simulink model "RLUb"  (R2018b)
settings: Solver=VariableStepAuto  StartTime=0.0  StopTime=15e-3  RelTol=1e-6  EnableMultiTasking=on
InitFcn:
  | RLUb_init
values from neighbouring files (symbols this model uses):
  D0 = Uout0 / Udc    [pmsm_control_init.m]
  Deadtime = 0e-6    (= 0)    [pmsm_control_init.m]
  dt = 50e-9    (= 5e-08)    [pmsm_init.m]
  fsw = 10e3    (= 10000)    [pmsm_control_init.m]
  I_FS = IabcFS / 0.8    [pmsm_control_init.m]
  L = Ld    [pmsm_control_init.m]    (also in pmsm_init.m = [Ld Lq])
  R = 18e-3    (= 0.018)    [pmsm_init.m]
  SampleMode = 1    [pmsm_control_init.m]
  U_FS = Udc / 0.8    [pmsm_control_init.m]
  Ub = Udc / 2    [pmsm_control_init.m]
  Udc = 300    [pmsm_init.m]
undefined symbols (not defined in the file or in its folder): A_I, A_P
libraries: powerlib x9, simulink x7
settings Model: ModifiedByFormat=The MathWorks Inc.  Creator=The MathWorks, Inc.  LastModifiedBy=The MathWorks Inc.
settings DataIOCC: LimitDataPoints=on  SaveFormat=Array  SaveOutput=off  SaveTime=off
settings OptimizationCC: ExpressionDepthLimit=2147483647  LifeSpan=1
settings DebuggingCC: MergeDetectMultiDrivingBlocksExec=none  SolverPrmCheckMsg=warning  FcnCallInpInsideContextMsg=warning  StateNameClashWarn=warning  SFUnexpectedBacktrackingDiag=warning  SFNoUnconditionalDefaultTransitionDiag=warning  SFExecutionAtInitializationDiag=none
settings HardwareCC: ProdBitPerPointer=32  ProdBitPerSizeT=32  ProdBitPerPtrDiffT=32  ProdLargestAtomicFloat=None  ProdIntDivRoundTo=Undefined  ProdEndianess=Unspecified  ProdWordSize=32  ProdHWDeviceType=32-bit Generic
settings ModelReferenceCC: PropagateSignalLabelsOutOfModel=off
settings SFSimCC: SimUseLocalCustomCode=off
settings RTWCC: RTWUseLocalCustomCode=off
settings CodeAppCC: StateflowObjectComments=on
settings GRTTargetCC: TargetLangStandard=C89/C90 (ANSI)  GeneratePreprocessorConditionals=Disable all  CombineOutputUpdateFcns=off  GRTInterface=on
settings ConfigComp: CovMetricSettings=dw  CovHtmlReporting=on  CovSaveCumulativeToWorkspaceVar=on  CovSaveSingleToWorkspaceVar=on  CovExternalEMLEnable=off  CovSFcnEnable=off

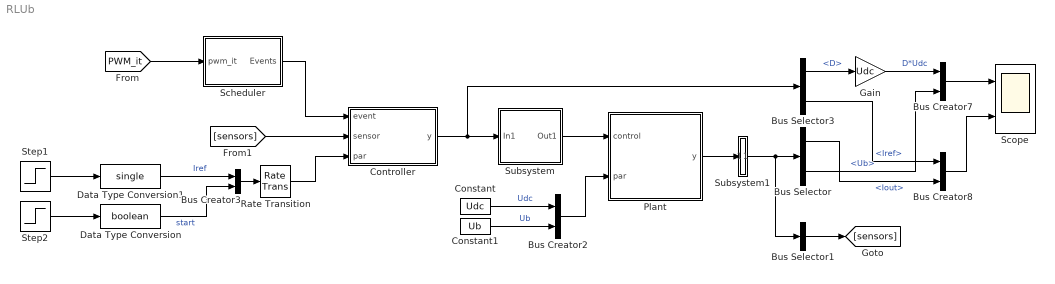
== system RLUb ==
  Bus Creator{2..3,7..8} (4 alike) : BusCreator  Inputs=2
  Bus Selector : BusSelector  OutputSignals=Iout,Ub
  Bus Selector1 : BusSelector  OutputSignals=Iout,Udc,Ub  OutputAsBus=on
  Bus Selector3 : BusSelector  OutputSignals=D,Iref
  Constant : Constant  Value=Udc  SampleTime=-1
  Constant1 : Constant  Value=Ub  SampleTime=-1
  Controller : Subsystem
  Data Type Conversion : DataTypeConversion  OutDataTypeStr=boolean
  Data Type Conversion1 : DataTypeConversion  OutDataTypeStr=single
  Gain : Gain  Gain=Udc
  Plant : Subsystem  Variant=on
  Rate Transition : RateTransition  Integrity=off  Deterministic=off
  Scheduler : Subsystem
  Scope : Scope  NumInputPorts=2
  Step1 : Step  Time=[7e-3]  After=10  SampleTime=0
  Step2 : Step  Time=[2e-3]  After=1e-3  SampleTime=0
  Subsystem : Subsystem
  Subsystem1 : Subsystem
  wires:
  Constant/1 -> Bus Creator2/1  "Udc"
  Constant1/1 -> Bus Creator2/2  "Ub"
  Bus Selector1/1 -> [sensors]
  Controller/1(y) -> Bus Selector3/1, Subsystem/1(In1)
  Bus Selector3/1 -> Gain/1  "<D>"
  Gain/1 -> Bus Creator7/1  "D*Udc"
  Bus Selector3/2 -> Bus Creator8/1  "<Iref>"
  Bus Selector/1 -> Bus Creator8/2  "<Iout>"
  Bus Creator7/1 -> Scope/1
  Bus Creator8/1 -> Scope/2
  Step1/1 -> Data Type Conversion1/1
  Scheduler/1(Events) -> Controller/1(event)
  Step2/1 -> Data Type Conversion/1
  Data Type Conversion/1 -> Bus Creator3/2  "start"
  Data Type Conversion1/1 -> Bus Creator3/1  "Iref"
  Bus Creator3/1 -> Rate Transition/1
  Plant/1(y) -> Subsystem1/1(In1)
  Bus Creator2/1 -> Plant/2(par)
  [sensors] -> Controller/2(sensor)
  Bus Selector/2 -> Bus Creator7/2  "<Ub>"
  Subsystem1/1(Out1) -> Bus Selector1/1, Bus Selector/1
  Rate Transition/1 -> Controller/3(par)
  [PWM_it] -> Scheduler/1(pwm_it)
  Subsystem/1(Out1) -> Plant/1(control)

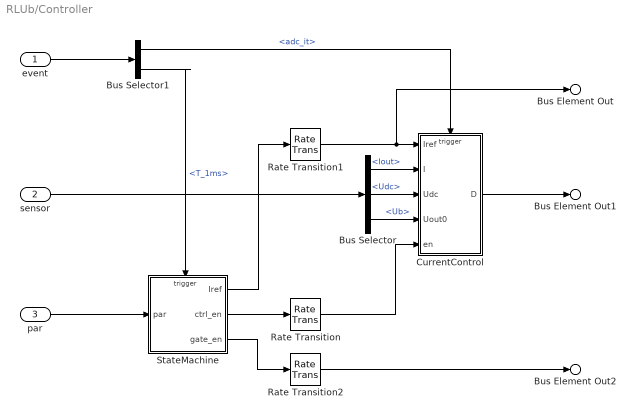
== system RLUb/Controller ==
  event : Inport
  sensor : Inport  Port=2
  par : Inport  Port=3
  Bus Selector : BusSelector  OutputSignals=Iout,Udc,Ub
  Bus Selector1 : BusSelector  OutputSignals=interrupts.adc_it,timers.T_1ms
  CurrentControl : Subsystem
  Rate Transition : RateTransition  Integrity=off  Deterministic=off
  Rate Transition1 : RateTransition  Integrity=off  Deterministic=off
  Rate Transition2 : RateTransition  Integrity=off  Deterministic=off
  StateMachine : Subsystem  TreatAsAtomicUnit=on
  Bus Element Out : Outport  PortName=y  Element=Iref
  Bus Element Out1 : Outport  PortName=y  Element=D
  Bus Element Out2 : Outport  PortName=y  Element=gate_en
  wires:
  StateMachine/1(Iref) -> Rate Transition1/1
  Rate Transition/1 -> CurrentControl/5(en)
  sensor/1 -> Bus Selector/1
  Bus Selector/1 -> CurrentControl/2(I)  "<Iout>"
  Bus Selector/2 -> CurrentControl/3(Udc)  "<Udc>"
  event/1 -> Bus Selector1/1
  Bus Selector1/1 -> CurrentControl/Trigger  "<adc_it>"
  CurrentControl/1(D) -> Bus Element Out1/1
  Bus Selector/3 -> CurrentControl/4(Uout0)  "<Ub>"
  Bus Selector1/2 -> StateMachine/Trigger  "<T_1ms>"
  StateMachine/2(ctrl_en) -> Rate Transition/1
  par/1 -> StateMachine/1(par)
  Rate Transition1/1 -> Bus Element Out/1, CurrentControl/1(Iref)
  StateMachine/3(gate_en) -> Rate Transition2/1
  Rate Transition2/1 -> Bus Element Out2/1

== system RLUb/Plant ==
  note: 1) Add Subsystem or Model blocks as valid variant choices.
      | 2) You cannot connect blocks at this level. At simulation, connectivity is automatically
      | determined, based on the active variant and port name matching.
  control : Inport
  par : Inport  Port=2
  RLUb_CT : Subsystem  VariantControl=PlantVariant == 11
  RLUb_DT : Subsystem  VariantControl=PlantVariant == 12
  RLUb_DTFX : Subsystem  VariantControl=PlantVariant == 13
  RLUb_SimPower : Subsystem  VariantControl=PlantVariant == 10
  y : Outport

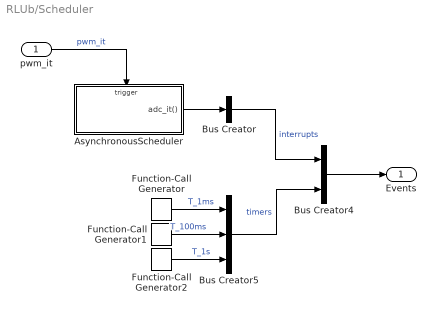
== system RLUb/Scheduler ==
  pwm_it : Inport
  AsynchronousScheduler : Stateflow chart  TreatAsAtomicUnit=on
      settings: RTWMemSecFuncInitTerm=Default  RTWMemSecFuncExecute=Default
  Bus Creator : BusCreator  Inputs=1
  Bus Creator4 : BusCreator  Inputs=2
  Bus Creator5 : BusCreator  Inputs=3
  Function-Call Generator : simulink/Ports & Subsystems/Function-Call Generator  sample_time=1e-3  numberOfIterations=1
  Function-Call Generator1 : simulink/Ports & Subsystems/Function-Call Generator  sample_time=100e-3  numberOfIterations=1
  Function-Call Generator2 : simulink/Ports & Subsystems/Function-Call Generator  sample_time=1  numberOfIterations=1
  Events : Outport
  wires:
  Bus Creator5/1 -> Bus Creator4/2  "timers"
  Function-Call Generator2/1 -> Bus Creator5/3  "T_1s"
  Bus Creator/1 -> Bus Creator4/1  "interrupts"
  pwm_it/1 -> AsynchronousScheduler/Trigger  "pwm_it"
  AsynchronousScheduler/1(adc_it()) -> Bus Creator/1
  Bus Creator4/1 -> Events/1
  Function-Call Generator1/1 -> Bus Creator5/2  "T_100ms"
  Function-Call Generator/1 -> Bus Creator5/1  "T_1ms"

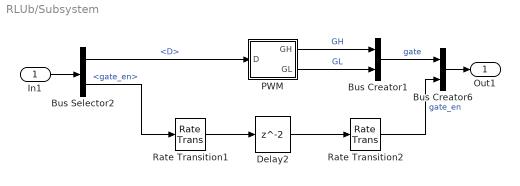
== system RLUb/Subsystem ==
  In1 : Inport
  Bus Creator1 : BusCreator  Inputs=2
  Bus Creator6 : BusCreator  Inputs=2
  Bus Selector2 : BusSelector  OutputSignals=D,gate_en
  Delay2 : Delay  InitialCondition=0
  PWM : Subsystem
  Rate Transition1 : RateTransition  Integrity=off  Deterministic=off  OutPortSampleTime=1e-3
  Rate Transition2 : RateTransition  Integrity=off  Deterministic=off
  Out1 : Outport
  wires:
  Rate Transition2/1 -> Bus Creator6/2  "gate_en"
  PWM/1(GH) -> Bus Creator1/1  "GH"
  Rate Transition1/1 -> Delay2/1
  Bus Selector2/1 -> PWM/1(D)  "<D>"
  Bus Selector2/2 -> Rate Transition1/1  "<gate_en>"
  Delay2/1 -> Rate Transition2/1
  In1/1 -> Bus Selector2/1
  PWM/2(GL) -> Bus Creator1/2  "GL"
  Bus Creator6/1 -> Out1/1
  Bus Creator1/1 -> Bus Creator6/1  "gate"

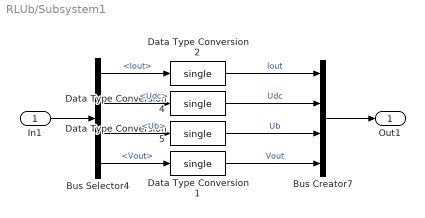
== system RLUb/Subsystem1 ==
  In1 : Inport
  Bus Creator7 : BusCreator  Inputs=4
  Bus Selector4 : BusSelector  OutputSignals=Iout,Udc,Ub,Vout
  Data Type Conversion{1..2,4..5} (4 alike) : DataTypeConversion  OutDataTypeStr=single
  Out1 : Outport
  wires:
  Data Type Conversion4/1 -> Bus Creator7/2  "Udc"
  Data Type Conversion2/1 -> Bus Creator7/1  "Iout"
  Bus Selector4/3 -> Data Type Conversion5/1  "<Ub>"
  Data Type Conversion5/1 -> Bus Creator7/3  "Ub"
  Bus Selector4/2 -> Data Type Conversion4/1  "<Udc>"
  Bus Selector4/1 -> Data Type Conversion2/1  "<Iout>"
  In1/1 -> Bus Selector4/1
  Bus Creator7/1 -> Out1/1
  Bus Selector4/4 -> Data Type Conversion1/1  "<Vout>"
  Data Type Conversion1/1 -> Bus Creator7/4  "Vout"

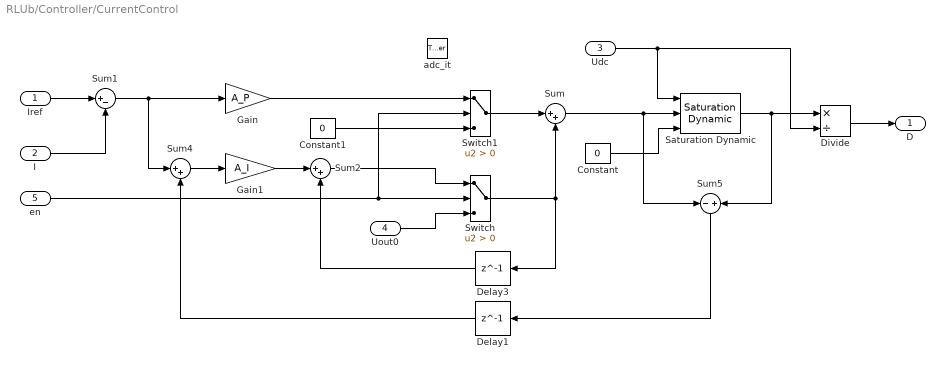
== system RLUb/Controller/CurrentControl ==
  Iref : Inport
  I : Inport  Port=2
  Udc : Inport  Port=3
  Uout0 : Inport  Port=4
  en : Inport  Port=5
  adc_it : TriggerPort  TriggerType=function-call  VariantControl=Variant  PortDimensions=1
  Constant : Constant  Value=0  OutDataTypeStr=Inherit: Inherit via back propagation  SampleTime=-1
  Constant1 : Constant  Value=0  OutDataTypeStr=Inherit: Inherit via back propagation  SampleTime=-1
  Delay1 : Delay  DelayLength=1  InitialCondition=0
  Delay3 : Delay  DelayLength=1  InitialCondition=0
  Divide : Product  Inputs=*/
  Gain : Gain  Gain=A_P
  Gain1 : Gain  Gain=A_I
  Saturation Dynamic : simulink/Discontinuities/Saturation Dynamic  OutMin=[]  OutMax=[]  OutDataTypeStr=Inherit: Same as second input  OutDataType=fixdt(1, 16)  OutScaling=2^-10  DoSatur=off
  Sum : Sum  Inputs=|++
  Sum1 : Sum  Inputs=|+-
  Sum2 : Sum  Inputs=|++
  Sum4 : Sum  Inputs=|++
  Sum5 : Sum  Inputs=-|+
  Switch : Switch  Criteria=u2 > Threshold
  Switch1 : Switch  Criteria=u2 > Threshold
  D : Outport
  wires:
  Divide/1 -> D/1
  Saturation Dynamic/1 -> Sum5/2, Divide/1
  Constant/1 -> Saturation Dynamic/3
  I/1 -> Sum1/2
  Udc/1 -> Divide/2, Saturation Dynamic/1
  Gain1/1 -> Sum2/1
  Iref/1 -> Sum1/1
  Uout0/1 -> Switch/3
  Sum4/1 -> Gain1/1
  Switch/1 -> Sum/2, Delay3/1
  Sum/1 -> Sum5/1, Saturation Dynamic/2
  Sum2/1 -> Switch/1
  Sum5/1 -> Delay1/1
  Sum1/1 -> Gain/1, Sum4/1
  Delay3/1 -> Sum2/2
  Delay1/1 -> Sum4/2
  Gain/1 -> Switch1/1
  Constant1/1 -> Switch1/3
  Switch1/1 -> Sum/1
  en/1 -> Switch1/2, Switch/2

== system RLUb/Controller/StateMachine ==
  par : Inport
  timer_1ms : TriggerPort  TriggerType=function-call  VariantControl=Variant
  Bus Selector2 : BusSelector  OutputSignals=Iref,start
  Delay1 : Delay  DelayLength=1  InitialCondition=0
  Delay2 : Delay  InitialCondition=0
  Iref : Outport
  ctrl_en : Outport  Port=2
  gate_en : Outport  Port=3
  wires:
  par/1 -> Delay1/1
  Bus Selector2/2 -> Delay2/1, gate_en/1  "<start>"
  Bus Selector2/1 -> Iref/1  "<Iref>"
  Delay1/1 -> Bus Selector2/1
  Delay2/1 -> ctrl_en/1

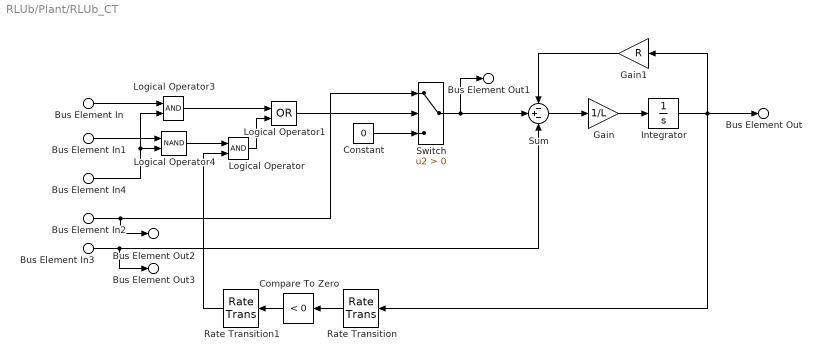
== system RLUb/Plant/RLUb_CT ==
  Bus Element In : Inport  PortName=control  Element=gate.GH
  Bus Element In1 : Inport  PortName=control  Element=gate.GL
  Bus Element In4 : Inport  PortName=control  Element=gate_en
  Bus Element In2 : Inport  Port=2  PortName=par  Element=Udc
  Bus Element In3 : Inport  Port=2  PortName=par  Element=Ub
  Compare To Zero : simulink/Logic and Bit Operations/Compare To Zero  relop=<  OutDataTypeStr=boolean
  Constant : Constant  Value=0  SampleTime=-1
  Gain : Gain  Gain=1/L
  Gain1 : Gain  Gain=R
  Integrator : Integrator
  Logical Operator : Logic  IconShape=distinctive  AllPortsSameDT=off  OutDataTypeStr=boolean
  Logical Operator1 : Logic  Operator=OR  IconShape=distinctive  AllPortsSameDT=off  OutDataTypeStr=boolean
  Logical Operator3 : Logic  IconShape=distinctive  AllPortsSameDT=off  OutDataTypeStr=boolean
  Logical Operator4 : Logic  Operator=NAND  IconShape=distinctive  AllPortsSameDT=off  OutDataTypeStr=boolean
  Rate Transition : RateTransition  OutPortSampleTime=1e-7
  Rate Transition1 : RateTransition
  Sum : Sum  Inputs=-+-
  Switch : Switch  Criteria=u2 > Threshold
  Bus Element Out : Outport  PortName=y  Element=Iout
  Bus Element Out1 : Outport  PortName=y  Element=Vout
  Bus Element Out2 : Outport  PortName=y  Element=Udc
  Bus Element Out3 : Outport  PortName=y  Element=Ub
  wires:
  Rate Transition/1 -> Compare To Zero/1
  Integrator/1 -> Rate Transition/1, Bus Element Out/1, Gain1/1
  Switch/1 -> Bus Element Out1/1, Sum/2
  Sum/1 -> Gain/1
  Gain/1 -> Integrator/1
  Gain1/1 -> Sum/1
  Bus Element In3/1 -> Bus Element Out3/1, Sum/3
  Bus Element In2/1 -> Bus Element Out2/1, Switch/1
  Constant/1 -> Switch/3
  Logical Operator3/1 -> Logical Operator1/1
  Logical Operator/1 -> Logical Operator1/2
  Logical Operator1/1 -> Switch/2
  Logical Operator4/1 -> Logical Operator/1
  Compare To Zero/1 -> Rate Transition1/1
  Rate Transition1/1 -> Logical Operator/2
  Bus Element In/1 -> Logical Operator3/1
  Bus Element In1/1 -> Logical Operator4/1
  Bus Element In4/1 -> Logical Operator3/2, Logical Operator4/2

== system RLUb/Plant/RLUb_DT ==
  control : Inport
  par : Inport  Port=2
  RLUb_DT : Subsystem  VariantControl=PlantVariant == 12
  Rate Transition : RateTransition  OutPortSampleTime=dt
  Rate Transition1 : RateTransition  OutPortSampleTime=dt
  Rate Transition2 : RateTransition
  y : Outport
  wires:
  control/1 -> Rate Transition/1
  RLUb_DT/1(y) -> Rate Transition2/1
  par/1 -> Rate Transition1/1
  Rate Transition/1 -> RLUb_DT/1(control)
  Rate Transition1/1 -> RLUb_DT/2(par)
  Rate Transition2/1 -> y/1

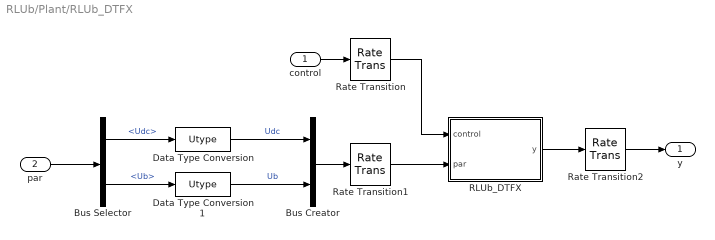
== system RLUb/Plant/RLUb_DTFX ==
  control : Inport
  par : Inport  Port=2
  Bus Creator : BusCreator  Inputs=2
  Bus Selector : BusSelector  OutputSignals=Udc,Ub
  Data Type Conversion : DataTypeConversion  OutDataTypeStr=Utype
  Data Type Conversion1 : DataTypeConversion  OutDataTypeStr=Utype
  RLUb_DTFX : Subsystem  VariantControl=PlantVariant == 12
  Rate Transition : RateTransition  OutPortSampleTime=dt
  Rate Transition1 : RateTransition  OutPortSampleTime=dt
  Rate Transition2 : RateTransition
  y : Outport
  wires:
  Rate Transition1/1 -> RLUb_DTFX/2(par)
  Rate Transition/1 -> RLUb_DTFX/1(control)
  RLUb_DTFX/1(y) -> Rate Transition2/1
  control/1 -> Rate Transition/1
  Rate Transition2/1 -> y/1
  Bus Creator/1 -> Rate Transition1/1
  Bus Selector/2 -> Data Type Conversion1/1  "<Ub>"
  par/1 -> Bus Selector/1
  Data Type Conversion/1 -> Bus Creator/1  "Udc"
  Bus Selector/1 -> Data Type Conversion/1  "<Udc>"
  Data Type Conversion1/1 -> Bus Creator/2  "Ub"

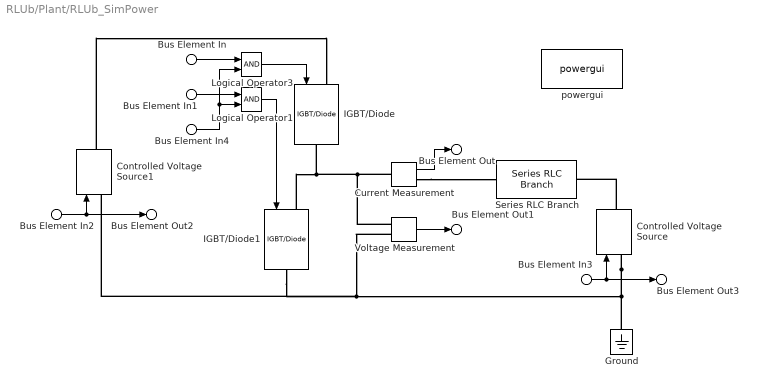
== system RLUb/Plant/RLUb_SimPower ==
  Bus Element In : Inport  PortName=control  Element=gate.GH
  Bus Element In1 : Inport  PortName=control  Element=gate.GL
  Bus Element In4 : Inport  PortName=control  Element=gate_en
  Bus Element In2 : Inport  Port=2  PortName=par  Element=Udc
  Bus Element In3 : Inport  Port=2  PortName=par  Element=Ub
  Controlled Voltage Source : powerlib/Electrical Sources/Controlled Voltage Source  Initialize=off  Source_Type=DC  Amplitude=0  Phase=0  Frequency=0  Measurements=None
  Controlled Voltage Source1 : powerlib/Electrical Sources/Controlled Voltage Source  Initialize=off  Source_Type=DC  Amplitude=0  Phase=0  Frequency=0  Measurements=None
  Current Measurement : powerlib/Measurements/Current Measurement  PhasorSimulation=off  OutputType=Complex  PSBequivalent=0
  Ground : powerlib/Elements/Ground  LConnTagsString=a
  IGBT/Diode : powerlib/Power Electronics/IGBT//Diode  Ron=1e-3  Rs=1e5  Cs=inf  Measurements=off
  IGBT/Diode1 : powerlib/Power Electronics/IGBT//Diode  Ron=1e-3  Rs=1e5  Cs=inf  Measurements=off
  Logical Operator1 : Logic  IconShape=distinctive  AllPortsSameDT=off  OutDataTypeStr=boolean
  Logical Operator3 : Logic  IconShape=distinctive  AllPortsSameDT=off  OutDataTypeStr=boolean
  Series RLC Branch : powerlib/Elements/Series RLC Branch  LConnTagsString=__new0  RConnTagsString=__new0  BranchType=RL  Resistance=R  Inductance=L  SetiL0=off  InitialCurrent=0  Capacitance=1e-6  Setx0=off  InitialVoltage=0  Measurements=None
  Voltage Measurement : powerlib/Measurements/Voltage Measurement  PhasorSimulation=off  OutputType=Complex  PSBequivalent=0
  powergui : powerlib/powergui  Priority=1  SimulationMode=Continuous  SampleTime=50e-6  frequency=60  Iterations=50  frequencyindice=0  Pbase=100e6  ErrMax=1e-4  UnitsV=kV  UnitsW=MW  buscounter=0  FunctionMessages=off  echomessages=off  EnableUseOfTLC=off  CurrentSourceSwitches=off  DisableSnubberDevices=off  DisableRonSwitches=off  DisableVfSwitches=off  DisplayEquations=off  SolverType=Tustin/Backward Euler (TBE)  Interpol=off  ExternalGateDelay=off  methode=off  Ts=100  x0status=blocks  SPID=on  SwTol=0  HookPort=off  RestoreLinks=warning  ResistiveCurrentMeasurement=off  Frange=[0:2:500]  Ylog=off  Xlog=on  ShowGrid=off  save=off  variable=ZData  structure=0  ZoomFFT=off  StartTime=0.0  cycles=1  DisplayStyle=1  fundamental=60  FreqAxis=off  MaxFrequency=1000  frequencyindicesteady=1  RmsSteady=1  display=off
  Bus Element Out : Outport  PortName=y  Element=Iout
  Bus Element Out1 : Outport  PortName=y  Element=Vout
  Bus Element Out2 : Outport  PortName=y  Element=Udc
  Bus Element Out3 : Outport  PortName=y  Element=Ub
  wires:
  Bus Element In2/1 -> Bus Element Out2/1, Controlled Voltage Source1/1
  Voltage Measurement/1 -> Bus Element Out1/1
  Current Measurement/1 -> Bus Element Out/1
  Bus Element In3/1 -> Controlled Voltage Source/1, Bus Element Out3/1
  Logical Operator1/1 -> IGBT/Diode1/1
  Logical Operator3/1 -> IGBT/Diode/1
  Bus Element In/1 -> Logical Operator3/1
  Bus Element In1/1 -> Logical Operator1/1
  Bus Element In4/1 -> Logical Operator1/2, Logical Operator3/2
  connections:
  Voltage Measurement/LConn1 -- Current Measurement/LConn1 -- IGBT/Diode1/LConn1 -- IGBT/Diode/RConn1
  Controlled Voltage Source/RConn1 -- Series RLC Branch/RConn1
  Controlled Voltage Source/LConn1 -- Ground/LConn1 -- Controlled Voltage Source1/LConn1 -- IGBT/Diode1/RConn1 -- Voltage Measurement/LConn2
  Controlled Voltage Source1/RConn1 -- IGBT/Diode/LConn1
  Current Measurement/RConn1 -- Series RLC Branch/LConn1

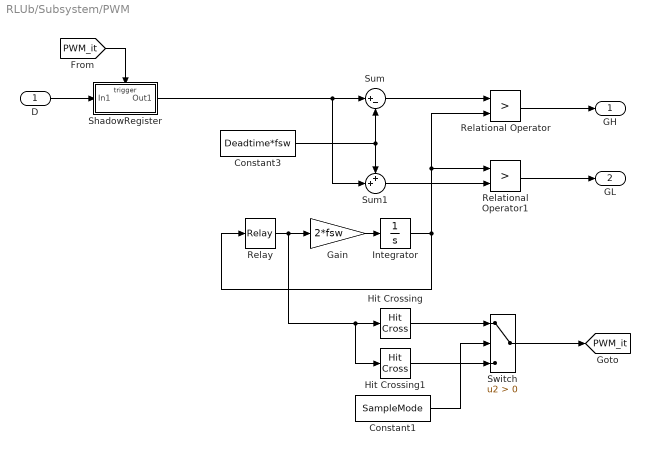
== system RLUb/Subsystem/PWM ==
  D : Inport
  Constant1 : Constant  Value=SampleMode  SampleTime=-1
  Constant3 : Constant  Value=Deadtime*fsw  SampleTime=-1
  Gain : Gain  Gain=2*fsw
  Hit Crossing : HitCross
  Hit Crossing1 : HitCross  HitCrossingDirection=rising
  Integrator : Integrator
  Relational Operator : RelationalOperator  Operator=>  OutDataTypeStr=boolean  RndMeth=Simplest
  Relational Operator1 : RelationalOperator  Operator=>  OutDataTypeStr=boolean  RndMeth=Simplest
  Relay : Relay  OnSwitchValue=1  OffSwitchValue=0  OnOutputValue=-1  OffOutputValue=1
  ShadowRegister : Subsystem
  Sum : Sum  Inputs=|+-
  Sum1 : Sum  Inputs=++|
  Switch : Switch  Criteria=u2 > Threshold
  GH : Outport
  GL : Outport  Port=2
  tag scope: PWM_it=global
  wires:
  Integrator/1 -> Relational Operator/2, Relational Operator1/1, Relay/1
  Gain/1 -> Integrator/1
  Relational Operator1/1 -> GL/1
  Relay/1 -> Hit Crossing1/1, Hit Crossing/1, Gain/1
  Constant3/1 -> Sum1/1, Sum/2
  Relational Operator/1 -> GH/1
  Sum1/1 -> Relational Operator1/2
  Sum/1 -> Relational Operator/1
  ShadowRegister/1(Out1) -> Sum1/2, Sum/1
  Hit Crossing/1 -> Switch/1
  Switch/1 -> [PWM_it]
  Hit Crossing1/1 -> Switch/3
  Constant1/1 -> Switch/2
  D/1 -> ShadowRegister/1(In1)
  [PWM_it] -> ShadowRegister/Trigger

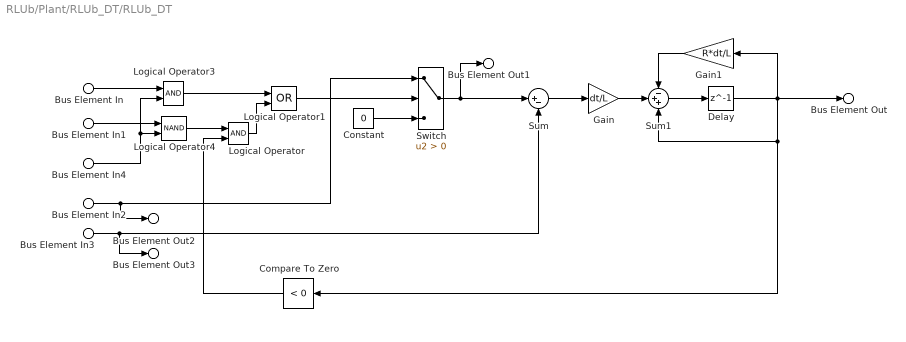
== system RLUb/Plant/RLUb_DT/RLUb_DT ==
  Bus Element In : Inport  PortName=control  Element=gate.GH
  Bus Element In1 : Inport  PortName=control  Element=gate.GL
  Bus Element In4 : Inport  PortName=control  Element=gate_en
  Bus Element In2 : Inport  Port=2  PortName=par  Element=Udc
  Bus Element In3 : Inport  Port=2  PortName=par  Element=Ub
  Compare To Zero : simulink/Logic and Bit Operations/Compare To Zero  relop=<  OutDataTypeStr=boolean
  Constant : Constant  Value=0  SampleTime=-1
  Delay : Delay  DelayLength=1
  Gain : Gain  Gain=dt/L
  Gain1 : Gain  Gain=R*dt/L
  Logical Operator : Logic  IconShape=distinctive  AllPortsSameDT=off  OutDataTypeStr=boolean
  Logical Operator1 : Logic  Operator=OR  IconShape=distinctive  AllPortsSameDT=off  OutDataTypeStr=boolean
  Logical Operator3 : Logic  IconShape=distinctive  AllPortsSameDT=off  OutDataTypeStr=boolean
  Logical Operator4 : Logic  Operator=NAND  IconShape=distinctive  AllPortsSameDT=off  OutDataTypeStr=boolean
  Sum : Sum  Inputs=|+-
  Sum1 : Sum  Inputs=-++
  Switch : Switch  Criteria=u2 > Threshold
  Bus Element Out : Outport  PortName=y  Element=Iout
  Bus Element Out1 : Outport  PortName=y  Element=Vout
  Bus Element Out2 : Outport  PortName=y  Element=Udc
  Bus Element Out3 : Outport  PortName=y  Element=Ub
  wires:
  Bus Element In4/1 -> Logical Operator4/2, Logical Operator3/2
  Bus Element In1/1 -> Logical Operator4/1
  Bus Element In/1 -> Logical Operator3/1
  Compare To Zero/1 -> Logical Operator/2
  Logical Operator4/1 -> Logical Operator/1
  Logical Operator1/1 -> Switch/2
  Logical Operator/1 -> Logical Operator1/2
  Logical Operator3/1 -> Logical Operator1/1
  Constant/1 -> Switch/3
  Bus Element In2/1 -> Switch/1, Bus Element Out2/1
  Bus Element In3/1 -> Sum/2, Bus Element Out3/1
  Gain1/1 -> Sum1/1
  Sum/1 -> Gain/1
  Switch/1 -> Sum/1, Bus Element Out1/1
  Delay/1 -> Bus Element Out/1, Gain1/1, Sum1/3, Compare To Zero/1
  Sum1/1 -> Delay/1
  Gain/1 -> Sum1/2

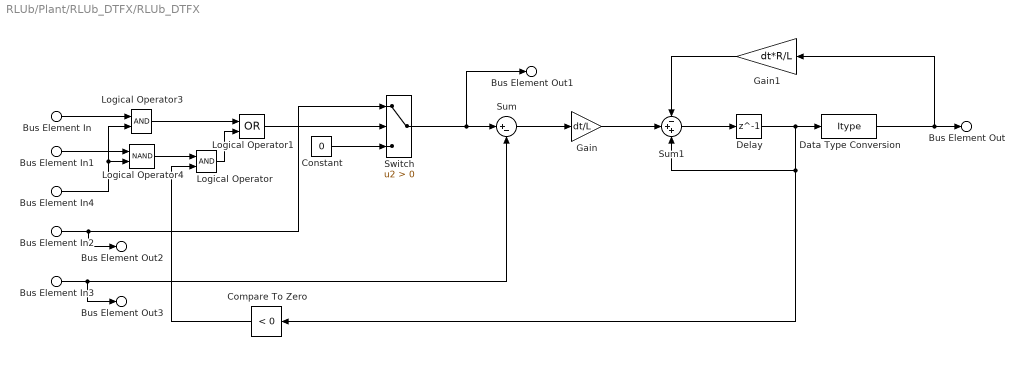
== system RLUb/Plant/RLUb_DTFX/RLUb_DTFX ==
  Bus Element In4 : Inport  PortName=control  Element=gate_en
  Bus Element In : Inport  PortName=control  Element=gate.GH
  Bus Element In1 : Inport  PortName=control  Element=gate.GL
  Bus Element In2 : Inport  Port=2  PortName=par  Element=Udc
  Bus Element In3 : Inport  Port=2  PortName=par  Element=Ub
  Compare To Zero : simulink/Logic and Bit Operations/Compare To Zero  relop=<  OutDataTypeStr=boolean
  Constant : Constant  Value=0  OutDataTypeStr=Inherit: Inherit via back propagation  SampleTime=-1
  Data Type Conversion : DataTypeConversion  OutDataTypeStr=Itype
  Delay : Delay  DelayLength=1
  Gain : Gain  Gain=dt/L  OutMax=[2*U_FS*dt/L]  OutDataTypeStr=fixdt(1,vbits)
  Gain1 : Gain  Gain=dt*R/L  OutMax=[I_FS*dt*R/L]  OutDataTypeStr=fixdt(1,vbits)
  Logical Operator : Logic  IconShape=distinctive  AllPortsSameDT=off  OutDataTypeStr=boolean
  Logical Operator1 : Logic  Operator=OR  IconShape=distinctive  AllPortsSameDT=off  OutDataTypeStr=boolean
  Logical Operator3 : Logic  IconShape=distinctive  AllPortsSameDT=off  OutDataTypeStr=boolean
  Logical Operator4 : Logic  Operator=NAND  IconShape=distinctive  AllPortsSameDT=off  OutDataTypeStr=boolean
  Sum : Sum  Inputs=|+-  OutDataTypeStr=Inherit: Same as accumulator
  Sum1 : Sum  Inputs=-++  OutMax=[I_FS*2]  OutDataTypeStr=fixdt(1,34+8)
  Switch : Switch  Criteria=u2 > Threshold
  Bus Element Out : Outport  PortName=y  Element=Iout
  Bus Element Out1 : Outport  PortName=y  Element=Vout
  Bus Element Out2 : Outport  PortName=y  Element=Udc
  Bus Element Out3 : Outport  PortName=y  Element=Ub
  wires:
  Sum1/1 -> Delay/1
  Delay/1 -> Data Type Conversion/1, Sum1/3, Compare To Zero/1
  Switch/1 -> Sum/1, Bus Element Out1/1
  Sum/1 -> Gain/1
  Gain1/1 -> Sum1/1
  Bus Element In3/1 -> Sum/2, Bus Element Out3/1
  Bus Element In2/1 -> Bus Element Out2/1, Switch/1
  Constant/1 -> Switch/3
  Logical Operator3/1 -> Logical Operator1/1
  Logical Operator/1 -> Logical Operator1/2
  Logical Operator1/1 -> Switch/2
  Logical Operator4/1 -> Logical Operator/1
  Compare To Zero/1 -> Logical Operator/2
  Bus Element In/1 -> Logical Operator3/1
  Bus Element In1/1 -> Logical Operator4/1
  Bus Element In4/1 -> Logical Operator3/2, Logical Operator4/2
  Data Type Conversion/1 -> Bus Element Out/1, Gain1/1
  Gain/1 -> Sum1/2

== system RLUb/Subsystem/PWM/ShadowRegister ==
  In1 : Inport  LatchByDelayingOutsideSignal=on
  Trigger : TriggerPort  VariantControl=Variant  PortDimensions=1
  Out1 : Outport  InitialOutput=[D0]
  wires:
  In1/1 -> Out1/1

== stateflow chart RLUb/Scheduler/AsynchronousScheduler ==
  settings: executeAtInitialization=1
  state AsynchronousScheduler
    AsynchronousScheduler -> (junction 6) : pwm_it { send(adc_it); }
  events: pwm_it input RISING_EDGE_EVENT; adc_it output FUNCTION_CALL_EVENT
